simulink model "smc"  (R2022b)
settings: Solver=ode45  StartTime=0.0  StopTime=20  RelTol=1e-4
undefined symbols (not defined in the file): m2
settings Model: Creator=Alex  LastModifiedBy=Alex

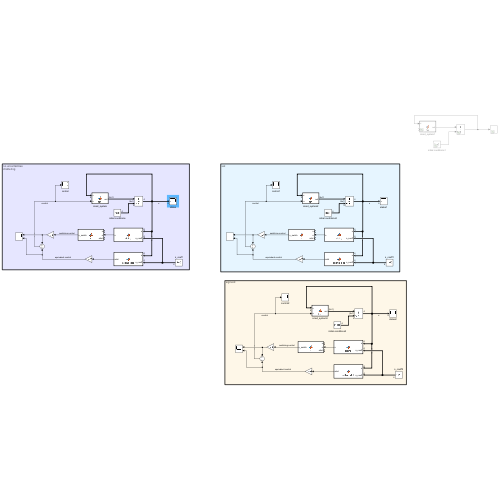
[thumbnail: Simulink's stored preview of the top-level diagram]
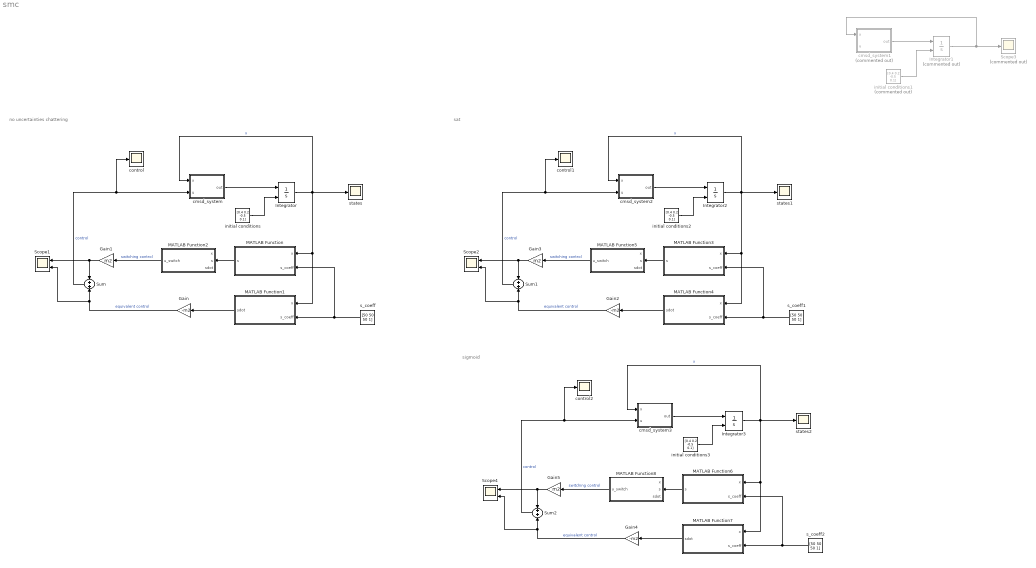
== system smc ==
  note: sigmoid
  note: sat
  note: no uncertainties
      | chattering
  Gain : Gain  Gain=-m2
  Gain1 : Gain  Gain=m2
  Gain2 : Gain  Gain=-m2
  Gain3 : Gain  Gain=m2
  Gain4 : Gain  Gain=-m2
  Gain5 : Gain  Gain=m2
  Integrator : Integrator  InitialConditionSource=external
  Integrator1 : Integrator  Commented=on  InitialConditionSource=external
  Integrator2 : Integrator  InitialConditionSource=external
  Integrator3 : Integrator  InitialConditionSource=external
  MATLAB Function : MATLAB Function  TreatAsAtomicUnit=on
  MATLAB Function1 : MATLAB Function  TreatAsAtomicUnit=on
  MATLAB Function2 : MATLAB Function  TreatAsAtomicUnit=on
  MATLAB Function3 : MATLAB Function  TreatAsAtomicUnit=on
  MATLAB Function4 : MATLAB Function  TreatAsAtomicUnit=on
  MATLAB Function5 : MATLAB Function  TreatAsAtomicUnit=on
  MATLAB Function6 : MATLAB Function  TreatAsAtomicUnit=on
  MATLAB Function7 : MATLAB Function  TreatAsAtomicUnit=on
  MATLAB Function8 : MATLAB Function  TreatAsAtomicUnit=on
  Scope1 : Scope  NumInputPorts=2
  Scope2 : Scope  NumInputPorts=2
  Scope3 : Scope  Commented=on
  Scope4 : Scope  NumInputPorts=2
  Sum : Sum
  Sum1 : Sum
  Sum2 : Sum
  cmsd_system : MATLAB Function  TreatAsAtomicUnit=on
  cmsd_system1 : MATLAB Function  Commented=on  TreatAsAtomicUnit=on
  cmsd_system2 : MATLAB Function  TreatAsAtomicUnit=on
  cmsd_system3 : MATLAB Function  TreatAsAtomicUnit=on
  control : Scope
  control1 : Scope
  control2 : Scope
  initial conditions : Constant  Value=[0.4 0.2 -0.5 0.1]
  initial conditions1 : Constant  Commented=on  Value=[0.4 0.2 -0.5 0.1]
  initial conditions2 : Constant  Value=[0.4 0.2 -0.5 0.1]
  initial conditions3 : Constant  Value=[0.4 0.2 -0.5 0.1]
  s_coeff : Constant  Value=[50 50 50 1]
  s_coeff1 : Constant  Value=[50 50 50 1]
  s_coeff2 : Constant  Value=[50 50 50 1]
  states : Scope
  states1 : Scope
  states2 : Scope
  wires:
  Integrator/1 -> MATLAB Function1/1(x), MATLAB Function/1(x), states/1, cmsd_system/1(x)  "x"
  initial conditions/1 -> Integrator/2
  s_coeff/1 -> MATLAB Function/2(s_coeff), MATLAB Function1/2(s_coeff)
  MATLAB Function1/1(sdot) -> Gain/1
  Gain/1 -> Scope1/2, Sum/2  "equivalent control"
  MATLAB Function/1(s) -> MATLAB Function2/2(s)
  MATLAB Function2/1(u_switch) -> Gain1/1  "switching control"
  Sum/1 -> cmsd_system/2(u), control/1  "control"
  cmsd_system/1(out) -> Integrator/1
  cmsd_system1/1(out) -> Integrator1/1
  initial conditions1/1 -> Integrator1/2
  Integrator1/1 -> cmsd_system1/1(x), Scope3/1
  Gain1/1 -> Sum/1, Scope1/1
  Gain3/1 -> Scope2/1, Sum1/1
  cmsd_system2/1(out) -> Integrator2/1
  Sum1/1 -> control1/1, cmsd_system2/2(u)  "control"
  MATLAB Function5/1(u_switch) -> Gain3/1  "switching control"
  MATLAB Function3/1(s) -> MATLAB Function5/2(s)
  Gain2/1 -> Sum1/2, Scope2/2  "equivalent control"
  MATLAB Function4/1(sdot) -> Gain2/1
  s_coeff1/1 -> MATLAB Function4/2(s_coeff), MATLAB Function3/2(s_coeff)
  initial conditions2/1 -> Integrator2/2
  Integrator2/1 -> cmsd_system2/1(x), states1/1, MATLAB Function3/1(x), MATLAB Function4/1(x)  "x"
  Integrator3/1 -> MATLAB Function7/1(x), MATLAB Function6/1(x), states2/1, cmsd_system3/1(x)  "x"
  initial conditions3/1 -> Integrator3/2
  s_coeff2/1 -> MATLAB Function6/2(s_coeff), MATLAB Function7/2(s_coeff)
  MATLAB Function7/1(sdot) -> Gain4/1
  Gain4/1 -> Scope4/2, Sum2/2  "equivalent control"
  MATLAB Function6/1(s) -> MATLAB Function8/2(s)
  MATLAB Function8/1(u_switch) -> Gain5/1  "switching control"
  Sum2/1 -> cmsd_system3/2(u), control2/1  "control"
  cmsd_system3/1(out) -> Integrator3/1
  Gain5/1 -> Sum2/1, Scope4/1

== matlab function smc/cmsd_system3 ==
  data: x input; u input; out output
function out = fcn(x,u)

k1=2/5; % N/m
k2=1;
m1=1; % kg
m2=2;
delta1=1/10; %Ns/m
delta2=1/5;
miu1=1/6; %
miu2=1/10;
g=[0 0 0 1/m2]';

xdot=[x(3);...
      x(4);...
      -delta1/m1*x(3)-k1/m1*x(1)+miu1/m1 * x(1)^3 - k2/m1 * (x(1)-x(2))+miu2/m1*(x(1)-x(2))^3;...
      -delta2/m2*x(4)-k2/m2*(x(2)-x(1))+miu2/m2*(x(2)-x(1))^3];



out= xdot+g*u;

== matlab function smc/MATLAB Function ==
  data: x input; s output; s_coeff input
function s = sliding(x,s_coeff)

s = s_coeff(1)*x(1)+s_coeff(2)*x(2)+s_coeff(3)*x(3)+s_coeff(4)*x(4);

== matlab function smc/MATLAB Function1 ==
  data: x input; sdot output; s_coeff input
function sdot = sliding_dot(x,s_coeff)
k1=2/5; % N/m
k2=1;
m1=1; % kg
m2=2;
delta1=1/10; %Ns/m
delta2=1/5;
miu1=1/6; %
miu2=1/10;
g=[0 0 0 1/m2]';

xdot=[x(3);...
      x(4);...
      -delta1/m1*x(3)-k1/m1*x(1)+miu1/m1 * x(1)^3 - k2/m1 * (x(1)-x(2))+miu2/m1*(x(1)-x(2))^3;...
      -delta2/m2*x(4)-k2/m2*(x(2)-x(1))+miu2/m2*(x(2)-x(1))^3];  % u is omitted here on purpose

sdot = s_coeff(1)*xdot(1)+s_coeff(2)*xdot(2)+s_coeff(3)*xdot(3)+s_coeff(4)*xdot(4);

== matlab function smc/MATLAB Function2 ==
  data: x input; s input; u_switch output; sdot input
function u_switch = v(x,s,sdot)

% k1=2/5; % N/m
% k2=1;
% m1=1; % kg
% m2=2;
% delta1=1/10; %
% delta2=1/5;
% miu1=1/6; %
% miu2=1/10;
L=1;
alpha=5;
u_switch = -(L+alpha/sqrt(2))*s/abs(s);

== matlab function smc/cmsd_system1 ==
  data: x input; u input; out output
function out = fcn(x,u)

k1=2/5; % N/m
k2=1;
m1=1; % kg
m2=20;
delta1=1/10; %Ns/m
delta2=1/5;
miu1=1/6; %
miu2=1/10;
g=[0 0 0 1/m2]';

xdot=[x(3);...
      x(4);...
      -delta1/m1*x(3)-k1/m1*x(1)+miu1/m1 * x(1)^3 - k2/m1 * (x(1)-x(2))+miu2/m1*(x(1)-x(2))^3;...
      -delta2/m2*x(4)-k2/m2*(x(2)-x(1))+miu2/m2*(x(2)-x(1))^3];



out= xdot+g*u;

== matlab function smc/MATLAB Function3 ==
  data: x input; s output; s_coeff input
function s = sliding(x,s_coeff)

s = s_coeff(1)*x(1)+s_coeff(2)*x(2)+s_coeff(3)*x(3)+s_coeff(4)*x(4);

== matlab function smc/MATLAB Function4 ==
  data: x input; sdot output; s_coeff input
function sdot = sliding_dot(x,s_coeff)
k1=2/5; % N/m
k2=1;
m1=1; % kg
m2=2;
delta1=1/10; %Ns/m
delta2=1/5;
miu1=1/6; %
miu2=1/10;
g=[0 0 0 1/m2]';

xdot=[x(3);...
      x(4);...
      -delta1/m1*x(3)-k1/m1*x(1)+miu1/m1 * x(1)^3 - k2/m1 * (x(1)-x(2))+miu2/m1*(x(1)-x(2))^3;...
      -delta2/m2*x(4)-k2/m2*(x(2)-x(1))+miu2/m2*(x(2)-x(1))^3];  % u is omitted here on purpose

sdot = s_coeff(1)*xdot(1)+s_coeff(2)*xdot(2)+s_coeff(3)*xdot(3)+s_coeff(4)*xdot(4);

== matlab function smc/MATLAB Function5 ==
  data: x input; s input; u_switch output; sdot input
function u_switch = v(x,s,sdot)

% k1=2/5; % N/m
% k2=1;
% m1=1; % kg
% m2=2;
% delta1=1/10; %
% delta2=1/5;
% miu1=1/6; %
% miu2=1/10;
L=1;
alpha=5;
miu=0.3;
u_switch = -(L+alpha/sqrt(2))*saturation_f(s/miu);


function out=saturation_f(x) 
    if(abs(x)<=1)
        out=x;
    else
        out=x/abs(x);
    end
end

end

== matlab function smc/cmsd_system2 ==
  data: x input; u input; out output
function out = fcn(x,u)

k1=2/5; % N/m
k2=1;
m1=1; % kg
m2=2;
delta1=1/10; %Ns/m
delta2=1/5;
miu1=1/6; %
miu2=1/10;
g=[0 0 0 1/m2]';

xdot=[x(3);...
      x(4);...
      -delta1/m1*x(3)-k1/m1*x(1)+miu1/m1 * x(1)^3 - k2/m1 * (x(1)-x(2))+miu2/m1*(x(1)-x(2))^3;...
      -delta2/m2*x(4)-k2/m2*(x(2)-x(1))+miu2/m2*(x(2)-x(1))^3];



out= xdot+g*u;

== matlab function smc/MATLAB Function6 ==
  data: x input; s output; s_coeff input
function s = sliding(x,s_coeff)

s = s_coeff(1)*x(1)+s_coeff(2)*x(2)+s_coeff(3)*x(3)+s_coeff(4)*x(4);

== matlab function smc/cmsd_system ==
  data: x input; u input; out output
function out = fcn(x,u)

k1=2/5; % N/m
k2=1;
m1=1; % kg
m2=2;
delta1=1/10; %Ns/m
delta2=1/5;
miu1=1/6; %
miu2=1/10;
g=[0 0 0 1/m2]';

xdot=[x(3);...
      x(4);...
      -delta1/m1*x(3)-k1/m1*x(1)+miu1/m1 * x(1)^3 - k2/m1 * (x(1)-x(2))+miu2/m1*(x(1)-x(2))^3;...
      -delta2/m2*x(4)-k2/m2*(x(2)-x(1))+miu2/m2*(x(2)-x(1))^3];



out= xdot+g*u;

== matlab function smc/MATLAB Function7 ==
  data: x input; sdot output; s_coeff input
function sdot = sliding_dot(x,s_coeff)
k1=2/5; % N/m
k2=1;
m1=1; % kg
m2=2;
delta1=1/10; %Ns/m
delta2=1/5;
miu1=1/6; %
miu2=1/10;
g=[0 0 0 1/m2]';

xdot=[x(3);...
      x(4);...
      -delta1/m1*x(3)-k1/m1*x(1)+miu1/m1 * x(1)^3 - k2/m1 * (x(1)-x(2))+miu2/m1*(x(1)-x(2))^3;...
      -delta2/m2*x(4)-k2/m2*(x(2)-x(1))+miu2/m2*(x(2)-x(1))^3];  % u is omitted here on purpose

sdot = s_coeff(1)*xdot(1)+s_coeff(2)*xdot(2)+s_coeff(3)*xdot(3)+s_coeff(4)*xdot(4);

== matlab function smc/MATLAB Function8 ==
  data: x input; s input; u_switch output; sdot input
function u_switch = v(x,s,sdot)

% k1=2/5; % N/m
% k2=1;
% m1=1; % kg
% m2=2;
% delta1=1/10; %
% delta2=1/5;
% miu1=1/6; %
% miu2=1/10;
L=1;
alpha=5;
eps=0.1;
u_switch = -(L+alpha/sqrt(2))*s/(abs(s)+eps);
